simulink library "amg_high_precision_rtc"  (R2015b)
settings: Solver=ode45  StartTime=0.0  StopTime=10.0  RelTol=1e-3
libraries: simulink x207, waijung_soft_i2c_lib x11, amg_high_precision_rtc x10
(part 5 of 5)

== system amg_high_precision_rtc/STM32F4/DS3231 Configure/Enabled Subsystem/Subsystem/Enabled Subsystem/Subsystem/Day count/Subsystem ==
  Month : Inport
  Year : Inport  Port=2
  Compare To Constant1 : simulink/Logic and Bit Operations/Compare To Constant  SystemSampleTime=-1  relop===  const=2  LogicOutDataTypeMode=uint8  ZeroCross=off
  Constant : Constant  Value=4  OutDataTypeStr=single
  Constant1 : Constant  Value=29  OutDataTypeStr=uint8
  Constant2 : Constant  Value=28  OutDataTypeStr=uint8
  Data Type Conversion : DataTypeConversion  OutDataTypeStr=single
  Data Type Conversion1 : DataTypeConversion  OutDataTypeStr=uint8
  Data Type Conversion2 : DataTypeConversion  OutDataTypeStr=uint8
  Data Type Conversion3 : DataTypeConversion  OutDataTypeStr=uint8
  Divide : Product  Inputs=*/
  Divide1 : Product  Inputs=**
  Subtract : Sum  Inputs=+-
  Switch : Switch  Criteria=u2 ~= 0
  Out1 : Outport
  Day count : Outport  Port=2
  wires:
  Month/1 -> Compare To Constant1/1
  Compare To Constant1/1 -> Out1/1
  Year/1 -> Data Type Conversion/1, Subtract/1
  Data Type Conversion/1 -> Divide/1
  Constant/1 -> Divide/2, Divide1/2
  Divide/1 -> Data Type Conversion1/1
  Subtract/1 -> Data Type Conversion2/1
  Constant1/1 -> Switch/3
  Constant2/1 -> Switch/1
  Switch/1 -> Day count/1
  Data Type Conversion2/1 -> Switch/2
  Data Type Conversion1/1 -> Divide1/1
  Divide1/1 -> Data Type Conversion3/1
  Data Type Conversion3/1 -> Subtract/2

== system amg_high_precision_rtc/Soft I2C/Soft-DS3231 Configure/Enabled Subsystem/Subsystem/Enabled Subsystem/Subsystem/Day count/Days 30 ==
  In1 : Inport
  Bitwise Operator : simulink/Logic and Bit Operations/Bitwise Operator  logicop=OR  UseBitMask=off  NumInputPorts=4  BitMask=bin2dec('11011001')  BitMaskRealWorld=Stored Integer
  Compare To Constant : simulink/Logic and Bit Operations/Compare To Constant  SystemSampleTime=-1  relop===  const=6  LogicOutDataTypeMode=uint8  ZeroCross=off
  Compare To Constant1 : simulink/Logic and Bit Operations/Compare To Constant  SystemSampleTime=-1  relop===  const=4  LogicOutDataTypeMode=uint8  ZeroCross=off
  Compare To Constant2 : simulink/Logic and Bit Operations/Compare To Constant  SystemSampleTime=-1  relop===  const=9  LogicOutDataTypeMode=uint8  ZeroCross=off
  Compare To Constant3 : simulink/Logic and Bit Operations/Compare To Constant  SystemSampleTime=-1  relop===  const=11  LogicOutDataTypeMode=uint8  ZeroCross=off
  Out1 : Outport
  wires:
  Bitwise Operator/1 -> Out1/1
  In1/1 -> Compare To Constant3/1, Compare To Constant2/1, Compare To Constant/1, Compare To Constant1/1
  Compare To Constant3/1 -> Bitwise Operator/4
  Compare To Constant2/1 -> Bitwise Operator/3
  Compare To Constant/1 -> Bitwise Operator/2
  Compare To Constant1/1 -> Bitwise Operator/1

== system amg_high_precision_rtc/Soft I2C/Soft-DS3231 Configure/Enabled Subsystem/Subsystem/Enabled Subsystem/Subsystem/Day count/Subsystem ==
  Month : Inport
  Year : Inport  Port=2
  Compare To Constant1 : simulink/Logic and Bit Operations/Compare To Constant  SystemSampleTime=-1  relop===  const=2  LogicOutDataTypeMode=uint8  ZeroCross=off
  Constant : Constant  Value=4  OutDataTypeStr=single
  Constant1 : Constant  Value=29  OutDataTypeStr=uint8
  Constant2 : Constant  Value=28  OutDataTypeStr=uint8
  Data Type Conversion : DataTypeConversion  OutDataTypeStr=single
  Data Type Conversion1 : DataTypeConversion  OutDataTypeStr=uint8
  Data Type Conversion2 : DataTypeConversion  OutDataTypeStr=uint8
  Data Type Conversion3 : DataTypeConversion  OutDataTypeStr=uint8
  Divide : Product  Inputs=*/
  Divide1 : Product  Inputs=**
  Subtract : Sum  Inputs=+-
  Switch : Switch  Criteria=u2 ~= 0
  Out1 : Outport
  Day count : Outport  Port=2
  wires:
  Data Type Conversion3/1 -> Subtract/2
  Divide1/1 -> Data Type Conversion3/1
  Data Type Conversion1/1 -> Divide1/1
  Data Type Conversion2/1 -> Switch/2
  Switch/1 -> Day count/1
  Constant2/1 -> Switch/1
  Constant1/1 -> Switch/3
  Subtract/1 -> Data Type Conversion2/1
  Divide/1 -> Data Type Conversion1/1
  Constant/1 -> Divide1/2, Divide/2
  Data Type Conversion/1 -> Divide/1
  Year/1 -> Subtract/1, Data Type Conversion/1
  Compare To Constant1/1 -> Out1/1
  Month/1 -> Compare To Constant1/1
